simulink model "problema2_simu"  (R2021b)
settings: Solver=VariableStepAuto  StartTime=0.0  StopTime=10.0  RelTol=1e-3
values from neighbouring files (symbols this model uses):
  A = [-1  0  0; -1  -2  -101; 1  1  0]    [matlab.mat]
  Ad = [0.990049833749  0  0; -0.0148301310913  0.975219702658  -0.998284581293; 0.00988400575538  0.00988400575538  0.994987714169]    [matlab.mat]    (also in problema1.m = double(Ad))
  B = [0  1; 1  -1; 0  0]    [matlab.mat]
  Bd = [0  0.00995016625083; 0.00988400575538  -0.00995016625083; 4.96265923899e-05  0]    [matlab.mat]    (also in problema1.m = double(Bd))
  C = [1 0 101]    [matlab.mat]
  Cd = [1 0 101]    [matlab.mat]    (also in problema1.m = C)
  D = [0 0]    [matlab.mat]
  Dd = [0 0]    [matlab.mat]    (also in problema1.m = D)
  den1z = [1 -2.96025725058 2.93080219879 -0.970445533549]    [matlab.mat]
  den2z = [1 -2.96025725058 2.93080219879 -0.970445533549]    [matlab.mat]
  h = 0.01    [matlab.mat]
  num1z = [0 0.00501228583138 1.6557894835e-05 -0.00492942906318]    [matlab.mat]
  num2z = [0 0.00995016625083 -0.019603891346 0.00975313975825]    [matlab.mat]
settings Model: Creator=laurentiu  LastModifiedBy=laurentiu

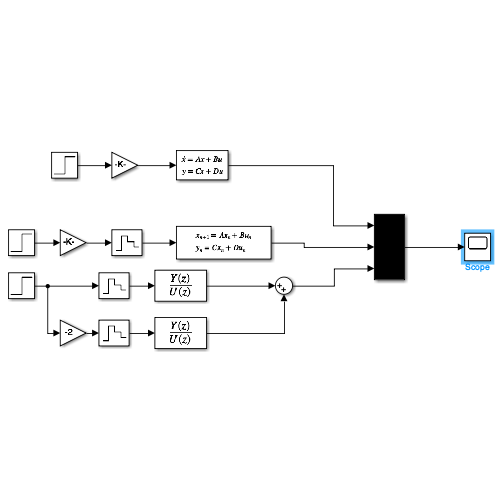
[thumbnail: Simulink's stored preview of the top-level diagram]
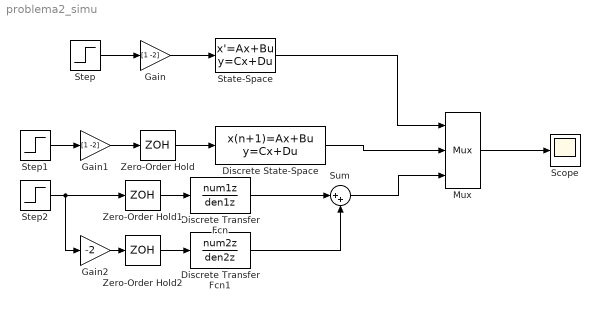
== system problema2_simu ==
  Discrete Transfer Fcn : DiscreteTransferFcn  Numerator=num1z  Denominator=den1z  SampleTime=h
  Discrete Transfer Fcn1 : DiscreteTransferFcn  Numerator=num2z  Denominator=den2z  SampleTime=h
  Discrete State-Space : DiscreteStateSpace  A=Ad  B=Bd  C=Cd  D=Dd  SampleTime=h
  Gain : Gain  Gain=[1 -2]
  Gain1 : Gain  Gain=[1 -2]
  Gain2 : Gain  Gain=-2
  Mux : Mux  Inputs=3
  Scope : Scope
  State-Space : StateSpace  A=A  B=B  C=C  D=D  InitialCondition=0
  Step : Step  SampleTime=0
  Step1 : Step  SampleTime=0
  Step2 : Step  SampleTime=0
  Sum : Sum  Inputs=|++
  Zero-Order Hold : ZeroOrderHold  SampleTime=h
  Zero-Order Hold1 : ZeroOrderHold  SampleTime=h
  Zero-Order Hold2 : ZeroOrderHold  SampleTime=h
  wires:
  Step/1 -> Gain/1
  Gain/1 -> State-Space/1
  Zero-Order Hold/1 -> Discrete State-Space/1
  State-Space/1 -> Mux/1
  Discrete State-Space/1 -> Mux/2
  Mux/1 -> Scope/1
  Step1/1 -> Gain1/1
  Gain1/1 -> Zero-Order Hold/1
  Step2/1 -> Zero-Order Hold1/1, Gain2/1
  Discrete Transfer Fcn/1 -> Sum/1
  Discrete Transfer Fcn1/1 -> Sum/2
  Sum/1 -> Mux/3
  Gain2/1 -> Zero-Order Hold2/1
  Zero-Order Hold2/1 -> Discrete Transfer Fcn1/1
  Zero-Order Hold1/1 -> Discrete Transfer Fcn/1
